simulink model "06.encoder"  (R2019b)
settings: Solver=FixedStepAuto  StartTime=0.0  StopTime=inf  FixedStep=1  MaxStep=1  RelTol=1e-3
settings Model: Creator=MARAT  LastModifiedBy=Marat
settings SFSimCC: CustomCodeUndefinedFunction=UseInterfaceOnly

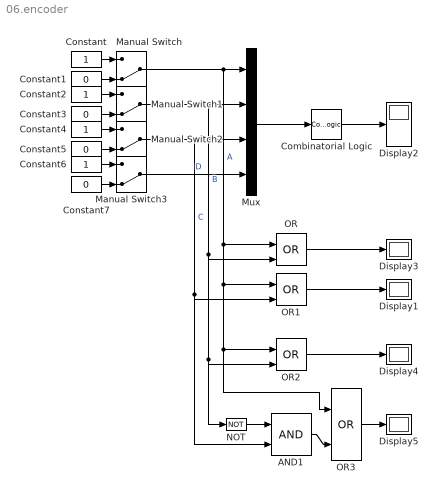
== system 06.encoder ==
  AND1 : Logic  IconShape=distinctive  AllPortsSameDT=off  OutDataTypeStr=boolean
  Combinatorial Logic : CombinatorialLogic  TruthTable=[0 0; 0 0; 0 1; 0 1; 1 0; 1 0; 1 0; 1 0; 1 1; 1 1; 1 1; 1 1; 1 1; 1 1; 1 1; 1 1]
  Constant{,2,4,6} (4 alike) : Constant  OutDataTypeStr=boolean
  Constant{1,3,5,7} (4 alike) : Constant  Value=0  OutDataTypeStr=boolean
  Display{1..5} (5 alike) : Display
  Manual Switch{,1..3} (4 alike) : ManualSwitch  CurrentSetting=0
  Mux : Mux
  NOT : Logic  Operator=NOT  IconShape=distinctive  AllPortsSameDT=off  OutDataTypeStr=boolean
  OR{,1..3} (4 alike) : Logic  Operator=OR  IconShape=distinctive  AllPortsSameDT=off  OutDataTypeStr=boolean
  wires:
  Mux/1 -> Combinatorial Logic/1
  Combinatorial Logic/1 -> Display2/1
  Constant/1 -> Manual Switch/1
  Constant1/1 -> Manual Switch/2
  Constant3/1 -> Manual Switch1/2
  Constant2/1 -> Manual Switch1/1
  Constant5/1 -> Manual Switch2/2
  Constant4/1 -> Manual Switch2/1
  OR/1 -> Display3/1
  Manual Switch/1 -> OR1/1, OR2/1, OR3/1, OR/1, Mux/1  "A"
  Manual Switch1/1 -> NOT/1, OR2/2, OR/2, Mux/2  "B"
  Manual Switch2/1 -> AND1/2, OR1/2, Mux/3  "C"
  Constant7/1 -> Manual Switch3/2
  Manual Switch3/1 -> Mux/4  "D"
  Constant6/1 -> Manual Switch3/1
  OR1/1 -> Display1/1
  OR2/1 -> Display4/1
  OR3/1 -> Display5/1
  AND1/1 -> OR3/2
  NOT/1 -> AND1/1
